simulink model "falownik"  (R2021b)
settings: Solver=ode1  StartTime=0.0  StopTime=1  FixedStep=0.00001  RelTol=1e-3
libraries: spsIGBTDiodeLib x6, spsAsynchronousMachineSIUnitsLib x1, spsDCVoltageSourceLib x1, slpidlib x1, spsSeriesRLCBranchLib x1, spsTriangleGeneratorLib x1, spsVoltageMeasurementLib x1, spspowerguiLib x1
settings Model: Creator=borutzki  LastModifiedBy=borutzki

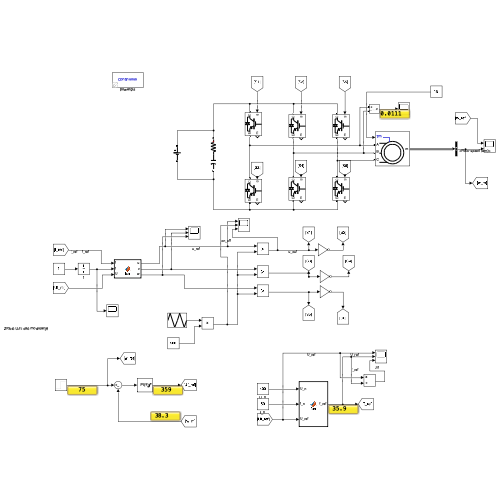
[thumbnail: Simulink's stored preview of the top-level diagram]
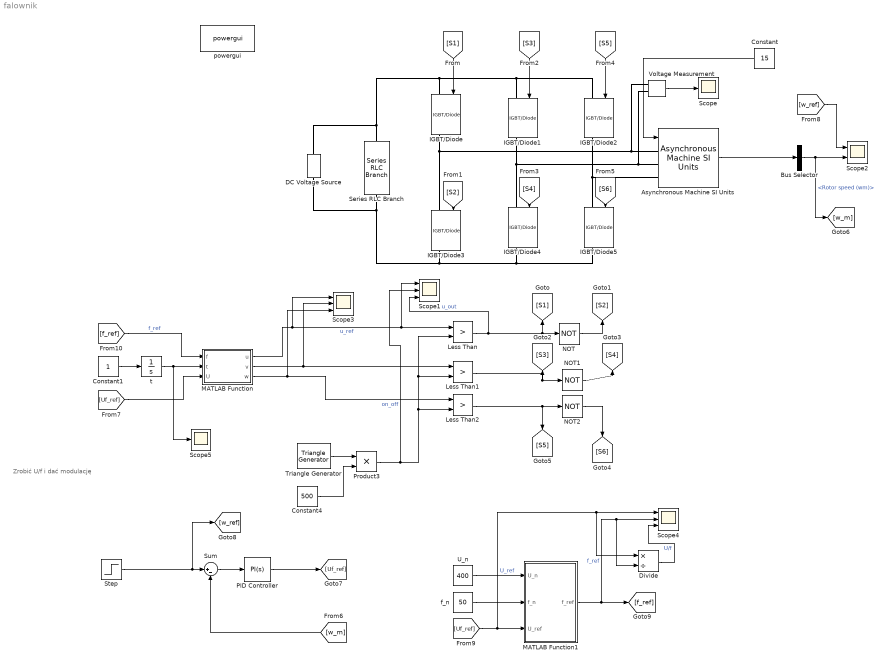
== system falownik ==
  note: Zrobić U/f i dać modulację
  Asynchronous Machine SI Units : spsAsynchronousMachineSIUnitsLib/Asynchronous Machine SI Units  RotorType=Squirrel-cage  PresetModel=No  MechanicalLoad=Torque Tm  ShowDetailedParameters=on  ReferenceFrame=Rotor  Units=SI  MeasurementBus=off  NominalParameters=[1.845e+04 400 50]  VoltageRatio=1  Stator=[0.5968 0.0003495]  Rotor=[0.6258 0.005473]  Cage1=[0.4155 0.002066]  Cage2=[0.4168 0.0003495]  Lm=0.0354  Mechanical=[0.05 0.005879 2]  PolePairs=2  InitialConditions=[0 0 0 0 0 0 0 0]  SimulateSaturation=off  Saturation=[14.03593122, 27.81365428, 53.79336849, 72.68890987, 97.98006896, 148.6815601, 215.7428561, 302.9841135, 428.7778367 ; 230, 322, 414, 460, 506, 552, 598, 644, 690]  LoadFlowParameters=1492000  TsPowergui=0  TsBlock=-1  IterativeModel=Trapezoidal non iterative  IterativeDiscreteModel=Trapezoidal non iterative  Pmec=1.492e+006
  Bus Selector : BusSelector  OutputSignals=Mechanical.Rotor speed (wm)
  Constant : Constant  Value=15
  Constant1 : Constant
  Constant4 : Constant  Value=500
  DC Voltage Source : spsDCVoltageSourceLib/DC Voltage Source  Amplitude=400  Measurements=None
  Divide : Product  Inputs=*/
  IGBT/Diode{,1..5} (6 alike) : spsIGBTDiodeLib/IGBT//Diode  Ron=1e-3  Rs=1e5  Cs=inf  Measurements=on
  Less Than : RelationalOperator  Operator=>  OutDataTypeStr=boolean  RndMeth=Simplest
  Less Than1 : RelationalOperator  Operator=>  OutDataTypeStr=boolean  RndMeth=Simplest
  Less Than2 : RelationalOperator  Operator=>  OutDataTypeStr=boolean  RndMeth=Simplest
  MATLAB Function : MATLAB Function  TreatAsAtomicUnit=on
  MATLAB Function1 : MATLAB Function  TreatAsAtomicUnit=on
  NOT : Logic  Operator=NOT  IconShape=distinctive  AllPortsSameDT=off  OutDataTypeStr=boolean
  NOT1 : Logic  Operator=NOT  IconShape=distinctive  AllPortsSameDT=off  OutDataTypeStr=boolean
  NOT2 : Logic  Operator=NOT  IconShape=distinctive  AllPortsSameDT=off  OutDataTypeStr=boolean
  PID Controller : slpidlib/PID Controller  Controller=PI  Form=Parallel  TimeDomain=Continuous-time  UseExternalTs=off  SampleTime=-1  IntegratorMethod=Forward Euler  FilterMethod=Forward Euler  ControllerParametersSource=internal  P=10  I=5  D=0  UseFilter=on  N=100  TunerSelectOption=Transfer Function Based (PID Tuner App)  InitialConditionSource=internal  InitialConditionForIntegrator=0  InitialConditionForFilter=0  DifferentiatorICPrevScaledInput=0  ExternalReset=none  TrackingMode=off  Kt=1  LimitOutput=on  SatLimitsSource=internal  UpperSaturationLimit=500  LowerSaturationLimit=0  LinearizeAsGain=on  AntiWindupMode=none  Kb=1  POutMin=[]  POutMax=[]  IOutMin=[]  IOutMax=[]  DOutMin=[]  DOutMax=[]  NOutMin=[]  NOutMax=[]  SumOutMin=[]  SumOutMax=[]  SaturationOutMin=[]  SaturationOutMax=[]  PParamMin=[]  PParamMax=[]  IParamMin=[]  IParamMax=[]  DParamMin=[]  DParamMax=[]  NParamMin=[]  NParamMax=[]  KbParamMin=[]  KbParamMax=[]  KtParamMin=[]  KtParamMax=[]  KbOutMin=[]  KbOutMax=[]  KtOutMin=[]  KtOutMax=[]  IntegratorOutMin=[]  IntegratorOutMax=[]  FilterOutMin=[]  FilterOutMax=[]  SumI1OutMin=[]  SumI1OutMax=[]  SumI2OutMin=[]  SumI2OutMax=[]  SumI3OutMin=[]  SumI3OutMax=[]  SumI4OutMin=[]  SumI4OutMax=[]  SumDOutMin=[]  SumDOutMax=[]  DifferentiatorOutMin=[]  DifferentiatorOutMax=[]  FilterDiffOutCoefMin=[]  FilterDiffOutCoefMax=[]  ReciprocalOutMin=[]  ReciprocalOutMax=[]  SumDenOutMin=[]  SumDenOutMax=[]  SumNumOutMin=[]  SumNumOutMax=[]  DivideOutMin=[]  DivideOutMax=[]  UdiffTsProdOutMin=[]  UdiffTsProdOutMax=[]  NTsProdOutMin=[]  NTsProdOutMax=[]  UintegralTsProdOutMin=[]  UintegralTsProdOutMax=[]  UngainTsProdOutMin=[]  UngainTsProdOutMax=[]  IntegratorContinuousStateAttributes=''  IntegratorStateMustResolveToSignalObject=off  IntegratorRTWStateStorageClass=Auto  FilterContinuousStateAttributes=''  FilterStateMustResolveToSignalObject=off  FilterRTWStateStorageClass=Auto  ParallelPVariant=InternalParameters  IdealPVariant=Disabled  IVariant=InternalParameters  DVariant=Disabled  IntegratorVariant=Continuous  SatVariant=Enabled  AWVariant=Passthrough  PCopyVariant=Disabled  TRVariant=Disabled  FdbkBlocksVariant=Forward  IdealPFdbkVariant=Disabled  SatFdbkVariant=Disabled  DerivativeFilterVariant=Disabled  NVariant=Disabled  NCopyVariant=Disabled_SignalSpec  FilterICVariant=Disabled  IntegratorICVariant=InternalICs  ExternalResetVariant=Disabled  TRSumVariant=Passthrough  SumFdbkVariant=Disabled  SumVariant=Sum_PI  TsampFilterVariant=InternalTs  TsampNgainVariant=Passthrough  TsampIntegralVariant=Passthrough  ExternalSaturationOutDataTypeStr=Inherit: Same as second input
  Product3 : Product
  Scope : Scope
  Scope1 : Scope  NumInputPorts=3
  Scope2 : Scope  NumInputPorts=2
  Scope3 : Scope  NumInputPorts=3
  Scope4 : Scope  NumInputPorts=3
  Scope5 : Scope
  Series RLC Branch : spsSeriesRLCBranchLib/Series RLC Branch  LConnTagsString=__new0  RConnTagsString=__new0  BranchType=RC  Resistance=0.001  Inductance=1e-3  SetiL0=off  InitialCurrent=0  Capacitance=600e-5  Setx0=off  InitialVoltage=0  Measurements=None
  Step : Step  Time=0.001  After=75  SampleTime=0
  Sum : Sum  Inputs=|+-
  Triangle Generator : spsTriangleGeneratorLib/Triangle Generator  Freq=5000  Phase=90  Ts=0
  U_n : Constant  Value=400
  Voltage Measurement : spsVoltageMeasurementLib/Voltage Measurement  PhasorSimulation=off  OutputType=Complex  PSBequivalent=0
  f_n : Constant  Value=50
  powergui : spspowerguiLib/powergui  Priority=1  SimulationMode=Continuous  SampleTime=5e-6  frequency=60  Iterations=50  frequencyindice=50  Pbase=100e6  ErrMax=1e-4  UnitsV=kV  UnitsW=MW  buscounter=0  FunctionMessages=off  echomessages=off  EnableUseOfTLC=off  CurrentSourceSwitches=off  DisableSnubberDevices=off  DisableRonSwitches=off  DisableVfSwitches=off  DisplayEquations=off  AutomaticDiscreteSolvers=off  SolverType=Tustin/Backward Euler (TBE)  Interpol=off  ExternalGateDelay=off  methode=off  Ts=100  x0status=blocks  SPID=on  SwTol=0  HookPort=off  NonlinearTolerance=1e-4  nMaxIteration=100  ContinueOnMaxIteration=off  RestoreLinks=warning  ResistiveCurrentMeasurement=off  Frange=[0:2:500]  Ylog=off  Xlog=on  ShowGrid=off  save=off  variable=ZData  structure=0  ZoomFFT=off  StartTime=0.0  cycles=1  DisplayStyle=1  fundamental=60  FreqAxis=off  MaxFrequency=1000  frequencyindicesteady=1  RmsSteady=1  display=off
  t : Integrator
  wires:
  MATLAB Function/1(u) -> Scope3/1, Scope1/1, Less Than/1  "u_ref"
  Product3/1 -> Less Than2/2, Less Than/2, Less Than1/2, Scope1/2  "on_off"
  Less Than/1 -> Scope1/3, NOT/1, [S1]  "u_out"
  NOT/1 -> [S2]
  Less Than1/1 -> NOT1/1, [S3]
  NOT1/1 -> [S4]
  Less Than2/1 -> NOT2/1, [S5]
  NOT2/1 -> [S6]
  [S1] -> IGBT/Diode/1
  [S2] -> IGBT/Diode3/1
  [S3] -> IGBT/Diode1/1
  [S4] -> IGBT/Diode4/1
  [S5] -> IGBT/Diode2/1
  [S6] -> IGBT/Diode5/1
  Voltage Measurement/1 -> Scope/1
  Asynchronous Machine SI Units/1 -> Bus Selector/1
  Bus Selector/1 -> [w_m], Scope2/2  "<Rotor speed (wm)>"
  MATLAB Function/2(v) -> Scope3/2, Less Than1/1
  MATLAB Function/3(w) -> Less Than2/1, Scope3/3
  Constant1/1 -> t/1
  t/1 -> Scope5/1, MATLAB Function/2(t)
  [f_ref] -> MATLAB Function/1(f)  "f_ref"
  [Uf_ref] -> MATLAB Function/3(U)
  Triangle Generator/1 -> Product3/1
  Constant4/1 -> Product3/2
  Step/1 -> [w_ref], Sum/1
  Sum/1 -> PID Controller/1
  [w_m] -> Sum/2
  PID Controller/1 -> [Uf_ref]
  [w_ref] -> Scope2/1
  f_n/1 -> MATLAB Function1/2(f_n)
  U_n/1 -> MATLAB Function1/1(U_n)
  [Uf_ref] -> Divide/1, Scope4/1, MATLAB Function1/3(U_ref)  "U_ref"
  MATLAB Function1/1(f_ref) -> Divide/2, Scope4/2, [f_ref]  "f_ref"
  Divide/1 -> Scope4/3  "U/f"
  Constant/1 -> Asynchronous Machine SI Units/1
  connections:
  Series RLC Branch/LConn1 -- DC Voltage Source/RConn1 -- IGBT/Diode/LConn1 -- IGBT/Diode2/LConn1 -- IGBT/Diode1/LConn1
  DC Voltage Source/LConn1 -- Series RLC Branch/RConn1 -- IGBT/Diode3/RConn1 -- IGBT/Diode5/RConn1 -- IGBT/Diode4/RConn1
  Asynchronous Machine SI Units/LConn1 -- Voltage Measurement/LConn1 -- IGBT/Diode3/LConn1 -- IGBT/Diode/RConn1
  IGBT/Diode4/LConn1 -- IGBT/Diode1/RConn1 -- Asynchronous Machine SI Units/LConn2 -- Voltage Measurement/LConn2
  Asynchronous Machine SI Units/LConn3 -- IGBT/Diode5/LConn1 -- IGBT/Diode2/RConn1

== matlab function falownik/MATLAB Function1 ==
  data: U_n input; f_ref output; f_n input; U_ref input
function f_ref = fcn(U_n,f_n,U_ref)
k = f_n/U_n
f_ref = abs(k*U_ref);

== matlab function falownik/MATLAB Function ==
  data: f input; u output; t input; U input; v output; w output
function [u,v,w]= fcn(f,t,U)

u = U*sin(2*pi*f*t);
v = U*sin(2*pi*f*t + 4*pi/3);
w = U*sin(2*pi*f*t + 2*pi/3);
